simulink model "fscsim"  (Simulink 5.1)
settings: Solver=ode45  SolverMode=SingleTasking  StartTime=0.0  StopTime=20e-3  MaxStep=Ts/10  RelTol=1e-3  AbsTol=1e-6
values from neighbouring files (symbols this model uses):
  Ts = PlantDataSeek.Ts    [seekdemo.m]
libraries: cstblocks x1
settings Model: LastModifiedBy=takeyori  LimitDataPoints=off  ProdHWDeviceType=Microprocessor  RTWOptions="-aEnforceIntegerDowncast=1 -aExtMode=0 -aExtModeTesting=0 -aFoldNonRolledExpr=1 -aForceParamTrailComments=0 -aGenerateComments=1 -aGenerateReport=0 -aIgnoreCustomStorageClasses=0 -aIncDataTypeInIds=0 -aIncHierarchyInIds=0 -aInlineInvariantSignals=1 -aInlinedPrmAccess=\"Literals\" -aLocalBlockOutputs=1 -aLogVarNameModifier=\"rt_\" -aMaxRTWIdLen=31 -aPrefixModelToSubsysFcnNames=1 -aRTWVerbose=1 -aRollThreshold=5 -aShowEliminatedStatements=0"

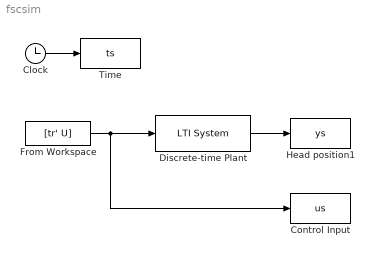
== system fscsim ==
  Clock : Clock
      settings: Decimation=10
  Control Input : ToWorkspace  VariableName=us  SampleTime=Ts/10  SaveFormat=Array
  Discrete-time Plant : cstblocks/LTI System  sys=sysd_P  IC=0
  From Workspace : FromWorkspace  VariableName=[tr' U]  SampleTime=Ts  Interpolate=off  OutputAfterFinalValue=Holding final value
  Head position1 : ToWorkspace  VariableName=ys  SampleTime=Ts/10  SaveFormat=Array
  Time : ToWorkspace  VariableName=ts  SampleTime=Ts/10  SaveFormat=Array
  wires:
  Clock/1 -> Time/1
  Discrete-time Plant/1 -> Head position1/1
  From Workspace/1 -> Control Input/1, Discrete-time Plant/1
